simulink model "Model"  (R2023b)
settings: Solver=FixedStepAuto  StartTime=0.0  StopTime=10  FixedStep=0.002  RelTol=1e-3
undefined symbols (not defined in the file or in its folder): K, X, Y, Z
libraries: sm_lib x47, nesl_utility x15, simulink x2, slpidlib x2
(part 3 of 4)

== matlab function Model/右腿VMC ==
  data: phi_1 input; phi_4 input; F input; T1 output; T2 output; Tp input
function [T1,T2]= fcn(phi_1,phi_4,F,Tp)

l_1=0.15;
l_2=0.27;
l_3=0.27;
l_4=0.15;
l_5=0.15;

J11=(2*(l_1*cos(phi_1) + (2*l_2*cos(2*atan(((4*l_2^2*(l_1*sin(phi_1) - l_4*sin(phi_4))^2 - ((l_1*sin(phi_1) - l_4*sin(phi_4))^2 + (l_5 - l_1*cos(phi_1) + l_4*cos(phi_4))^2 + l_2^2 - l_3^2)^2 + 4*l_2^2*(l_5 - l_1*cos(phi_1) + l_4*cos(phi_4))^2)^(1/2) - 2*l_2*(l_1*sin(phi_1) - l_4*sin(phi_4)))/((l_1*sin(phi_1) - l_4*sin(phi_4))^2 + (l_5 - l_1*cos(phi_1) + l_4*cos(phi_4))^2 + l_2^2 - l_3^2 + 2*l_2*(l_5 - l_1*cos(phi_1) + l_4*cos(phi_4)))))*(((8*l_1*l_2^2*cos(phi_1)*(l_1*sin(phi_1) - l_4*sin(phi_4)) - 2*(2*l_1*cos(phi_1)*(l_1*sin(phi_1) - l_4*sin(phi_4)) + 2*l_1*sin(phi_1)*(l_5 - l_1*cos(phi_1) + l_4*cos(phi_4)))*((l_1*sin(phi_1) - l_4*sin(phi_4))^2 + (l_5 - l_1*cos(phi_1) + l_4*cos(phi_4))^2 + l_2^2 - l_3^2) + 8*l_1*l_2^2*sin(phi_1)*(l_5 - l_1*cos(phi_1) + l_4*cos(phi_4)))/(2*(4*l_2^2*(l_1*sin(phi_1) - l_4*sin(phi_4))^2 - ((l_1*sin(phi_1) - l_4*sin(phi_4))^2 + (l_5 - l_1*cos(phi_1) + l_4*cos(phi_4))^2 + l_2^2 - l_3^2)^2 + 4*l_2^2*(l_5 - l_1*cos(phi_1) + l_4*cos(phi_4))^2)^(1/2)) - 2*l_1*l_2*cos(phi_1))/((l_1*sin(phi_1) - l_4*sin(phi_4))^2 + (l_5 - l_1*cos(phi_1) + l_4*cos(phi_4))^2 + l_2^2 - l_3^2 + 2*l_2*(l_5 - l_1*cos(phi_1) + l_4*cos(phi_4))) - (((4*l_2^2*(l_1*sin(phi_1) - l_4*sin(phi_4))^2 - ((l_1*sin(phi_1) - l_4*sin(phi_4))^2 + (l_5 - l_1*cos(phi_1) + l_4*cos(phi_4))^2 + l_2^2 - l_3^2)^2 + 4*l_2^2*(l_5 - l_1*cos(phi_1) + l_4*cos(phi_4))^2)^(1/2) - 2*l_2*(l_1*sin(phi_1) - l_4*sin(phi_4)))*(2*l_1*l_2*sin(phi_1) + 2*l_1*cos(phi_1)*(l_1*sin(phi_1) - l_4*sin(phi_4)) + 2*l_1*sin(phi_1)*(l_5 - l_1*cos(phi_1) + l_4*cos(phi_4))))/((l_1*sin(phi_1) - l_4*sin(phi_4))^2 + (l_5 - l_1*cos(phi_1) + l_4*cos(phi_4))^2 + l_2^2 - l_3^2 + 2*l_2*(l_5 - l_1*cos(phi_1) + l_4*cos(phi_4)))^2))/(((4*l_2^2*(l_1*sin(phi_1) - l_4*sin(phi_4))^2 - ((l_1*sin(phi_1) - l_4*sin(phi_4))^2 + (l_5 - l_1*cos(phi_1) + l_4*cos(phi_4))^2 + l_2^2 - l_3^2)^2 + 4*l_2^2*(l_5 - l_1*cos(phi_1) + l_4*cos(phi_4))^2)^(1/2) - 2*l_2*(l_1*sin(phi_1) - l_4*sin(phi_4)))^2/((l_1*sin(phi_1) - l_4*sin(phi_4))^2 + (l_5 - l_1*cos(phi_1) + l_4*cos(phi_4))^2 + l_2^2 - l_3^2 + 2*l_2*(l_5 - l_1*cos(phi_1) + l_4*cos(phi_4)))^2 + 1))*(l_2*sin(2*atan(((4*l_2^2*(l_1*sin(phi_1) - l_4*sin(phi_4))^2 - ((l_1*sin(phi_1) - l_4*sin(phi_4))^2 + (l_5 - l_1*cos(phi_1) + l_4*cos(phi_4))^2 + l_2^2 - l_3^2)^2 + 4*l_2^2*(l_5 - l_1*cos(phi_1) + l_4*cos(phi_4))^2)^(1/2) - 2*l_2*(l_1*sin(phi_1) - l_4*sin(phi_4)))/((l_1*sin(phi_1) - l_4*sin(phi_4))^2 + (l_5 - l_1*cos(phi_1) + l_4*cos(phi_4))^2 + l_2^2 - l_3^2 + 2*l_2*(l_5 - l_1*cos(phi_1) + l_4*cos(phi_4))))) + l_1*sin(phi_1)) - 2*(l_1*sin(phi_1) + (2*l_2*sin(2*atan(((4*l_2^2*(l_1*sin(phi_1) - l_4*sin(phi_4))^2 - ((l_1*sin(phi_1) - l_4*sin(phi_4))^2 + (l_5 - l_1*cos(phi_1) + l_4*cos(phi_4))^2 + l_2^2 - l_3^2)^2 + 4*l_2^2*(l_5 - l_1*cos(phi_1) + l_4*cos(phi_4))^2)^(1/2) - 2*l_2*(l_1*sin(phi_1) - l_4*sin(phi_4)))/((l_1*sin(phi_1) - l_4*sin(phi_4))^2 + (l_5 - l_1*cos(phi_1) + l_4*cos(phi_4))^2 + l_2^2 - l_3^2 + 2*l_2*(l_5 - l_1*cos(phi_1) + l_4*cos(phi_4)))))*(((8*l_1*l_2^2*cos(phi_1)*(l_1*sin(phi_1) - l_4*sin(phi_4)) - 2*(2*l_1*cos(phi_1)*(l_1*sin(phi_1) - l_4*sin(phi_4)) + 2*l_1*sin(phi_1)*(l_5 - l_1*cos(phi_1) + l_4*cos(phi_4)))*((l_1*sin(phi_1) - l_4*sin(phi_4))^2 + (l_5 - l_1*cos(phi_1) + l_4*cos(phi_4))^2 + l_2^2 - l_3^2) + 8*l_1*l_2^2*sin(phi_1)*(l_5 - l_1*cos(phi_1) + l_4*cos(phi_4)))/(2*(4*l_2^2*(l_1*sin(phi_1) - l_4*sin(phi_4))^2 - ((l_1*sin(phi_1) - l_4*sin(phi_4))^2 + (l_5 - l_1*cos(phi_1) + l_4*cos(phi_4))^2 + l_2^2 - l_3^2)^2 + 4*l_2^2*(l_5 - l_1*cos(phi_1) + l_4*cos(phi_4))^2)^(1/2)) - 2*l_1*l_2*cos(phi_1))/((l_1*sin(phi_1) - l_4*sin(phi_4))^2 + (l_5 - l_1*cos(phi_1) + l_4*cos(phi_4))^2 + l_2^2 - l_3^2 + 2*l_2*(l_5 - l_1*cos(phi_1) + l_4*cos(phi_4))) - (((4*l_2^2*(l_1*sin(phi_1) - l_4*sin(phi_4))^2 - ((l_1*sin(phi_1) - l_4*sin(phi_4))^2 + (l_5 - l_1*cos(phi_1) + l_4*cos(phi_4))^2 + l_2^2 - l_3^2)^2 + 4*l_2^2*(l_5 - l_1*cos(phi_1) + l_4*cos(phi_4))^2)^(1/2) - 2*l_2*(l_1*sin(phi_1) - l_4*sin(phi_4)))*(2*l_1*l_2*sin(phi_1) + 2*l_1*cos(phi_1)*(l_1*sin(phi_1) - l_4*sin(phi_4)) + 2*l_1*sin(phi_1)*(l_5 - l_1*cos(phi_1) + l_4*cos(phi_4))))/((l_1*sin(phi_1) - l_4*sin(phi_4))^2 + (l_5 - l_1*cos(phi_1) + l_4*cos(phi_4))^2 + l_2^2 - l_3^2 + 2*l_2*(l_5 - l_1*cos(phi_1) + l_4*cos(phi_4)))^2))/(((4*l_2^2*(l_1*sin(phi_1) - l_4*sin(phi_4))^2 - ((l_1*sin(phi_1) - l_4*sin(phi_4))^2 + (l_5 - l_1*cos(phi_1) + l_4*cos(phi_4))^2 + l_2^2 - l_3^2)^2 + 4*l_2^2*(l_5 - l_1*cos(phi_1) + l_4*cos(phi_4))^2)^(1/2) - 2*l_2*(l_1*sin(phi_1) - l_4*sin(phi_4)))^2/((l_1*sin(phi_1) - l_4*sin(phi_4))^2 + (l_5 - l_1*cos(phi_1) + l_4*cos(phi_4))^2 + l_2^2 - l_3^2 + 2*l_2*(l_5 - l_1*cos(phi_1) + l_4*cos(phi_4)))^2 + 1))*(l_2*cos(2*atan(((4*l_2^2*(l_1*sin(phi_1) - l_4*sin(phi_4))^2 - ((l_1*sin(phi_1) - l_4*sin(phi_4))^2 + (l_5 - l_1*cos(phi_1) + l_4*cos(phi_4))^2 + l_2^2 - l_3^2)^2 + 4*l_2^2*(l_5 - l_1*cos(phi_1) + l_4*cos(phi_4))^2)^(1/2) - 2*l_2*(l_1*sin(phi_1) - l_4*sin(phi_4)))/((l_1*sin(phi_1) - l_4*sin(phi_4))^2 + (l_5 - l_1*cos(phi_1) + l_4*cos(phi_4))^2 + l_2^2 - l_3^2 + 2*l_2*(l_5 - l_1*cos(phi_1) + l_4*cos(phi_4))))) - l_5/2 + l_1*cos(phi_1)))/(2*((l_2*sin(2*atan(((4*l_2^2*(l_1*sin(phi_1) - l_4*sin(phi_4))^2 - ((l_1*sin(phi_1) - l_4*sin(phi_4))^2 + (l_5 - l_1*cos(phi_1) + l_4*cos(phi_4))^2 + l_2^2 - l_3^2)^2 + 4*l_2^2*(l_5 - l_1*cos(phi_1) + l_4*cos(phi_4))^2)^(1/2) - 2*l_2*(l_1*sin(phi_1) - l_4*sin(phi_4)))/((l_1*sin(phi_1) - l_4*sin(phi_4))^2 + (l_5 - l_1*cos(phi_1) + l_4*cos(phi_4))^2 + l_2^2 - l_3^2 + 2*l_2*(l_5 - l_1*cos(phi_1) + l_4*cos(phi_4))))) + l_1*sin(phi_1))^2 + (l_2*cos(2*atan(((4*l_2^2*(l_1*sin(phi_1) - l_4*sin(phi_4))^2 - ((l_1*sin(phi_1) - l_4*sin(phi_4))^2 + (l_5 - l_1*cos(phi_1) + l_4*cos(phi_4))^2 + l_2^2 - l_3^2)^2 + 4*l_2^2*(l_5 - l_1*cos(phi_1) + l_4*cos(phi_4))^2)^(1/2) - 2*l_2*(l_1*sin(phi_1) - l_4*sin(phi_4)))/((l_1*sin(phi_1) - l_4*sin(phi_4))^2 + (l_5 - l_1*cos(phi_1) + l_4*cos(phi_4))^2 + l_2^2 - l_3^2 + 2*l_2*(l_5 - l_1*cos(phi_1) + l_4*cos(phi_4))))) - l_5/2 + l_1*cos(phi_1))^2)^(1/2));
J12=((4*l_2*sin(2*atan(((4*l_2^2*(l_1*sin(phi_1) - l_4*sin(phi_4))^2 - ((l_1*sin(phi_1) - l_4*sin(phi_4))^2 + (l_5 - l_1*cos(phi_1) + l_4*cos(phi_4))^2 + l_2^2 - l_3^2)^2 + 4*l_2^2*(l_5 - l_1*cos(phi_1) + l_4*cos(phi_4))^2)^(1/2) - 2*l_2*(l_1*sin(phi_1) - l_4*sin(phi_4)))/((l_1*sin(phi_1) - l_4*sin(phi_4))^2 + (l_5 - l_1*cos(phi_1) + l_4*cos(phi_4))^2 + l_2^2 - l_3^2 + 2*l_2*(l_5 - l_1*cos(phi_1) + l_4*cos(phi_4)))))*(((8*l_2^2*l_4*cos(phi_4)*(l_1*sin(phi_1) - l_4*sin(phi_4)) - 2*(2*l_4*cos(phi_4)*(l_1*sin(phi_1) - l_4*sin(phi_4)) + 2*l_4*sin(phi_4)*(l_5 - l_1*cos(phi_1) + l_4*cos(phi_4)))*((l_1*sin(phi_1) - l_4*sin(phi_4))^2 + (l_5 - l_1*cos(phi_1) + l_4*cos(phi_4))^2 + l_2^2 - l_3^2) + 8*l_2^2*l_4*sin(phi_4)*(l_5 - l_1*cos(phi_1) + l_4*cos(phi_4)))/(2*(4*l_2^2*(l_1*sin(phi_1) - l_4*sin(phi_4))^2 - ((l_1*sin(phi_1) - l_4*sin(phi_4))^2 + (l_5 - l_1*cos(phi_1) + l_4*cos(phi_4))^2 + l_2^2 - l_3^2)^2 + 4*l_2^2*(l_5 - l_1*cos(phi_1) + l_4*cos(phi_4))^2)^(1/2)) - 2*l_2*l_4*cos(phi_4))/((l_1*sin(phi_1) - l_4*sin(phi_4))^2 + (l_5 - l_1*cos(phi_1) + l_4*cos(phi_4))^2 + l_2^2 - l_3^2 + 2*l_2*(l_5 - l_1*cos(phi_1) + l_4*cos(phi_4))) - (((4*l_2^2*(l_1*sin(phi_1) - l_4*sin(phi_4))^2 - ((l_1*sin(phi_1) - l_4*sin(phi_4))^2 + (l_5 - l_1*cos(phi_1) + l_4*cos(phi_4))^2 + l_2^2 - l_3^2)^2 + 4*l_2^2*(l_5 - l_1*cos(phi_1) + l_4*cos(phi_4))^2)^(1/2) - 2*l_2*(l_1*sin(phi_1) - l_4*sin(phi_4)))*(2*l_2*l_4*sin(phi_4) + 2*l_4*cos(phi_4)*(l_1*sin(phi_1) - l_4*sin(phi_4)) + 2*l_4*sin(phi_4)*(l_5 - l_1*cos(phi_1) + l_4*cos(phi_4))))/((l_1*sin(phi_1) - l_4*sin(phi_4))^2 + (l_5 - l_1*cos(phi_1) + l_4*cos(phi_4))^2 + l_2^2 - l_3^2 + 2*l_2*(l_5 - l_1*cos(phi_1) + l_4*cos(phi_4)))^2)*(l_2*cos(2*atan(((4*l_2^2*(l_1*sin(phi_1) - l_4*sin(phi_4))^2 - ((l_1*sin(phi_1) - l_4*sin(phi_4))^2 + (l_5 - l_1*cos(phi_1) + l_4*cos(phi_4))^2 + l_2^2 - l_3^2)^2 + 4*l_2^2*(l_5 - l_1*cos(phi_1) + l_4*cos(phi_4))^2)^(1/2) - 2*l_2*(l_1*sin(phi_1) - l_4*sin(phi_4)))/((l_1*sin(phi_1) - l_4*sin(phi_4))^2 + (l_5 - l_1*cos(phi_1) + l_4*cos(phi_4))^2 + l_2^2 - l_3^2 + 2*l_2*(l_5 - l_1*cos(phi_1) + l_4*cos(phi_4))))) - l_5/2 + l_1*cos(phi_1)))/(((4*l_2^2*(l_1*sin(phi_1) - l_4*sin(phi_4))^2 - ((l_1*sin(phi_1) - l_4*sin(phi_4))^2 + (l_5 - l_1*cos(phi_1) + l_4*cos(phi_4))^2 + l_2^2 - l_3^2)^2 + 4*l_2^2*(l_5 - l_1*cos(phi_1) + l_4*cos(phi_4))^2)^(1/2) - 2*l_2*(l_1*sin(phi_1) - l_4*sin(phi_4)))^2/((l_1*sin(phi_1) - l_4*sin(phi_4))^2 + (l_5 - l_1*cos(phi_1) + l_4*cos(phi_4))^2 + l_2^2 - l_3^2 + 2*l_2*(l_5 - l_1*cos(phi_1) + l_4*cos(phi_4)))^2 + 1) - (4*l_2*cos(2*atan(((4*l_2^2*(l_1*sin(phi_1) - l_4*sin(phi_4))^2 - ((l_1*sin(phi_1) - l_4*sin(phi_4))^2 + (l_5 - l_1*cos(phi_1) + l_4*cos(phi_4))^2 + l_2^2 - l_3^2)^2 + 4*l_2^2*(l_5 - l_1*cos(phi_1) + l_4*cos(phi_4))^2)^(1/2) - 2*l_2*(l_1*sin(phi_1) - l_4*sin(phi_4)))/((l_1*sin(phi_1) - l_4*sin(phi_4))^2 + (l_5 - l_1*cos(phi_1) + l_4*cos(phi_4))^2 + l_2^2 - l_3^2 + 2*l_2*(l_5 - l_1*cos(phi_1) + l_4*cos(phi_4)))))*(l_2*sin(2*atan(((4*l_2^2*(l_1*sin(phi_1) - l_4*sin(phi_4))^2 - ((l_1*sin(phi_1) - l_4*sin(phi_4))^2 + (l_5 - l_1*cos(phi_1) + l_4*cos(phi_4))^2 + l_2^2 - l_3^2)^2 + 4*l_2^2*(l_5 - l_1*cos(phi_1) + l_4*cos(phi_4))^2)^(1/2) - 2*l_2*(l_1*sin(phi_1) - l_4*sin(phi_4)))/((l_1*sin(phi_1) - l_4*sin(phi_4))^2 + (l_5 - l_1*cos(phi_1) + l_4*cos(phi_4))^2 + l_2^2 - l_3^2 + 2*l_2*(l_5 - l_1*cos(phi_1) + l_4*cos(phi_4))))) + l_1*sin(phi_1))*(((8*l_2^2*l_4*cos(phi_4)*(l_1*sin(phi_1) - l_4*sin(phi_4)) - 2*(2*l_4*cos(phi_4)*(l_1*sin(phi_1) - l_4*sin(phi_4)) + 2*l_4*sin(phi_4)*(l_5 - l_1*cos(phi_1) + l_4*cos(phi_4)))*((l_1*sin(phi_1) - l_4*sin(phi_4))^2 + (l_5 - l_1*cos(phi_1) + l_4*cos(phi_4))^2 + l_2^2 - l_3^2) + 8*l_2^2*l_4*sin(phi_4)*(l_5 - l_1*cos(phi_1) + l_4*cos(phi_4)))/(2*(4*l_2^2*(l_1*sin(phi_1) - l_4*sin(phi_4))^2 - ((l_1*sin(phi_1) - l_4*sin(phi_4))^2 + (l_5 - l_1*cos(phi_1) + l_4*cos(phi_4))^2 + l_2^2 - l_3^2)^2 + 4*l_2^2*(l_5 - l_1*cos(phi_1) + l_4*cos(phi_4))^2)^(1/2)) - 2*l_2*l_4*cos(phi_4))/((l_1*sin(phi_1) - l_4*sin(phi_4))^2 + (l_5 - l_1*cos(phi_1) + l_4*cos(phi_4))^2 + l_2^2 - l_3^2 + 2*l_2*(l_5 - l_1*cos(phi_1) + l_4*cos(phi_4))) - (((4*l_2^2*(l_1*sin(phi_1) - l_4*sin(phi_4))^2 - ((l_1*sin(phi_1) - l_4*sin(phi_4))^2 + (l_5 - l_1*cos(phi_1) + l_4*cos(phi_4))^2 + l_2^2 - l_3^2)^2 + 4*l_2^2*(l_5 - l_1*cos(phi_1) + l_4*cos(phi_4))^2)^(1/2) - 2*l_2*(l_1*sin(phi_1) - l_4*sin(phi_4)))*(2*l_2*l_4*sin(phi_4) + 2*l_4*cos(phi_4)*(l_1*sin(phi_1) - l_4*sin(phi_4)) + 2*l_4*sin(phi_4)*(l_5 - l_1*cos(phi_1) + l_4*cos(phi_4))))/((l_1*sin(phi_1) - l_4*sin(phi_4))^2 + (l_5 - l_1*cos(phi_1) + l_4*cos(phi_4))^2 + l_2^2 - l_3^2 + 2*l_2*(l_5 - l_1*cos(phi_1) + l_4*cos(phi_4)))^2))/(((4*l_2^2*(l_1*sin(phi_1) - l_4*sin(phi_4))^2 - ((l_1*sin(phi_1) - l_4*sin(phi_4))^2 + (l_5 - l_1*cos(phi_1) + l_4*cos(phi_4))^2 + l_2^2 - l_3^2)^2 + 4*l_2^2*(l_5 - l_1*cos(phi_1) + l_4*cos(phi_4))^2)^(1/2) - 2*l_2*(l_1*sin(phi_1) - l_4*sin(phi_4)))^2/((l_1*sin(phi_1) - l_4*sin(phi_4))^2 + (l_5 - l_1*cos(phi_1) + l_4*cos(phi_4))^2 + l_2^2 - l_3^2 + 2*l_2*(l_5 - l_1*cos(phi_1) + l_4*cos(phi_4)))^2 + 1))/(2*((l_2*sin(2*atan(((4*l_2^2*(l_1*sin(phi_1) - l_4*sin(phi_4))^2 - ((l_1*sin(phi_1) - l_4*sin(phi_4))^2 + (l_5 - l_1*cos(phi_1) + l_4*cos(phi_4))^2 + l_2^2 - l_3^2)^2 + 4*l_2^2*(l_5 - l_1*cos(phi_1) + l_4*cos(phi_4))^2)^(1/2) - 2*l_2*(l_1*sin(phi_1) - l_4*sin(phi_4)))/((l_1*sin(phi_1) - l_4*sin(phi_4))^2 + (l_5 - l_1*cos(phi_1) + l_4*cos(phi_4))^2 + l_2^2 - l_3^2 + 2*l_2*(l_5 - l_1*cos(phi_1) + l_4*cos(phi_4))))) + l_1*sin(phi_1))^2 + (l_2*cos(2*atan(((4*l_2^2*(l_1*sin(phi_1) - l_4*sin(phi_4))^2 - ((l_1*sin(phi_1) - l_4*sin(phi_4))^2 + (l_5 - l_1*cos(phi_1) + l_4*cos(phi_4))^2 + l_2^2 - l_3^2)^2 + 4*l_2^2*(l_5 - l_1*cos(phi_1) + l_4*cos(phi_4))^2)^(1/2) - 2*l_2*(l_1*sin(phi_1) - l_4*sin(phi_4)))/((l_1*sin(phi_1) - l_4*sin(phi_4))^2 + (l_5 - l_1*cos(phi_1) + l_4*cos(phi_4))^2 + l_2^2 - l_3^2 + 2*l_2*(l_5 - l_1*cos(phi_1) + l_4*cos(phi_4))))) - l_5/2 + l_1*cos(phi_1))^2)^(1/2));
J21=((l_1*sin(phi_1) + (2*l_2*sin(2*atan(((4*l_2^2*(l_1*sin(phi_1) - l_4*sin(phi_4))^2 - ((l_1*sin(phi_1) - l_4*sin(phi_4))^2 + (l_5 - l_1*cos(phi_1) + l_4*cos(phi_4))^2 + l_2^2 - l_3^2)^2 + 4*l_2^2*(l_5 - l_1*cos(phi_1) + l_4*cos(phi_4))^2)^(1/2) - 2*l_2*(l_1*sin(phi_1) - l_4*sin(phi_4)))/((l_1*sin(phi_1) - l_4*sin(phi_4))^2 + (l_5 - l_1*cos(phi_1) + l_4*cos(phi_4))^2 + l_2^2 - l_3^2 + 2*l_2*(l_5 - l_1*cos(phi_1) + l_4*cos(phi_4)))))*(((8*l_1*l_2^2*cos(phi_1)*(l_1*sin(phi_1) - l_4*sin(phi_4)) - 2*(2*l_1*cos(phi_1)*(l_1*sin(phi_1) - l_4*sin(phi_4)) + 2*l_1*sin(phi_1)*(l_5 - l_1*cos(phi_1) + l_4*cos(phi_4)))*((l_1*sin(phi_1) - l_4*sin(phi_4))^2 + (l_5 - l_1*cos(phi_1) + l_4*cos(phi_4))^2 + l_2^2 - l_3^2) + 8*l_1*l_2^2*sin(phi_1)*(l_5 - l_1*cos(phi_1) + l_4*cos(phi_4)))/(2*(4*l_2^2*(l_1*sin(phi_1) - l_4*sin(phi_4))^2 - ((l_1*sin(phi_1) - l_4*sin(phi_4))^2 + (l_5 - l_1*cos(phi_1) + l_4*cos(phi_4))^2 + l_2^2 - l_3^2)^2 + 4*l_2^2*(l_5 - l_1*cos(phi_1) + l_4*cos(phi_4))^2)^(1/2)) - 2*l_1*l_2*cos(phi_1))/((l_1*sin(phi_1) - l_4*sin(phi_4))^2 + (l_5 - l_1*cos(phi_1) + l_4*cos(phi_4))^2 + l_2^2 - l_3^2 + 2*l_2*(l_5 - l_1*cos(phi_1) + l_4*cos(phi_4))) - (((4*l_2^2*(l_1*sin(phi_1) - l_4*sin(phi_4))^2 - ((l_1*sin(phi_1) - l_4*sin(phi_4))^2 + (l_5 - l_1*cos(phi_1) + l_4*cos(phi_4))^2 + l_2^2 - l_3^2)^2 + 4*l_2^2*(l_5 - l_1*cos(phi_1) + l_4*cos(phi_4))^2)^(1/2) - 2*l_2*(l_1*sin(phi_1) - l_4*sin(phi_4)))*(2*l_1*l_2*sin(phi_1) + 2*l_1*cos(phi_1)*(l_1*sin(phi_1) - l_4*sin(phi_4)) + 2*l_1*sin(phi_1)*(l_5 - l_1*cos(phi_1) + l_4*cos(phi_4))))/((l_1*sin(phi_1) - l_4*sin(phi_4))^2 + (l_5 - l_1*cos(phi_1) + l_4*cos(phi_4))^2 + l_2^2 - l_3^2 + 2*l_2*(l_5 - l_1*cos(phi_1) + l_4*cos(phi_4)))^2))/(((4*l_2^2*(l_1*sin(phi_1) - l_4*sin(phi_4))^2 - ((l_1*sin(phi_1) - l_4*sin(phi_4))^2 + (l_5 - l_1*cos(phi_1) + l_4*cos(phi_4))^2 + l_2^2 - l_3^2)^2 + 4*l_2^2*(l_5 - l_1*cos(phi_1) + l_4*cos(phi_4))^2)^(1/2) - 2*l_2*(l_1*sin(phi_1) - l_4*sin(phi_4)))^2/((l_1*sin(phi_1) - l_4*sin(phi_4))^2 + (l_5 - l_1*cos(phi_1) + l_4*cos(phi_4))^2 + l_2^2 - l_3^2 + 2*l_2*(l_5 - l_1*cos(phi_1) + l_4*cos(phi_4)))^2 + 1))/((l_2*sin(2*atan(((4*l_2^2*(l_1*sin(phi_1) - l_4*sin(phi_4))^2 - ((l_1*sin(phi_1) - l_4*sin(phi_4))^2 + (l_5 - l_1*cos(phi_1) + l_4*cos(phi_4))^2 + l_2^2 - l_3^2)^2 + 4*l_2^2*(l_5 - l_1*cos(phi_1) + l_4*cos(phi_4))^2)^(1/2) - 2*l_2*(l_1*sin(phi_1) - l_4*sin(phi_4)))/((l_1*sin(phi_1) - l_4*sin(phi_4))^2 + (l_5 - l_1*cos(phi_1) + l_4*cos(phi_4))^2 + l_2^2 - l_3^2 + 2*l_2*(l_5 - l_1*cos(phi_1) + l_4*cos(phi_4))))) + l_1*sin(phi_1))^2 + (l_2*cos(2*atan(((4*l_2^2*(l_1*sin(phi_1) - l_4*sin(phi_4))^2 - ((l_1*sin(phi_1) - l_4*sin(phi_4))^2 + (l_5 - l_1*cos(phi_1) + l_4*cos(phi_4))^2 + l_2^2 - l_3^2)^2 + 4*l_2^2*(l_5 - l_1*cos(phi_1) + l_4*cos(phi_4))^2)^(1/2) - 2*l_2*(l_1*sin(phi_1) - l_4*sin(phi_4)))/((l_1*sin(phi_1) - l_4*sin(phi_4))^2 + (l_5 - l_1*cos(phi_1) + l_4*cos(phi_4))^2 + l_2^2 - l_3^2 + 2*l_2*(l_5 - l_1*cos(phi_1) + l_4*cos(phi_4))))) - l_5/2 + l_1*cos(phi_1))^2)^(1/2) + ((2*(l_1*cos(phi_1) + (2*l_2*cos(2*atan(((4*l_2^2*(l_1*sin(phi_1) - l_4*sin(phi_4))^2 - ((l_1*sin(phi_1) - l_4*sin(phi_4))^2 + (l_5 - l_1*cos(phi_1) + l_4*cos(phi_4))^2 + l_2^2 - l_3^2)^2 + 4*l_2^2*(l_5 - l_1*cos(phi_1) + l_4*cos(phi_4))^2)^(1/2) - 2*l_2*(l_1*sin(phi_1) - l_4*sin(phi_4)))/((l_1*sin(phi_1) - l_4*sin(phi_4))^2 + (l_5 - l_1*cos(phi_1) + l_4*cos(phi_4))^2 + l_2^2 - l_3^2 + 2*l_2*(l_5 - l_1*cos(phi_1) + l_4*cos(phi_4)))))*(((8*l_1*l_2^2*cos(phi_1)*(l_1*sin(phi_1) - l_4*sin(phi_4)) - 2*(2*l_1*cos(phi_1)*(l_1*sin(phi_1) - l_4*sin(phi_4)) + 2*l_1*sin(phi_1)*(l_5 - l_1*cos(phi_1) + l_4*cos(phi_4)))*((l_1*sin(phi_1) - l_4*sin(phi_4))^2 + (l_5 - l_1*cos(phi_1) + l_4*cos(phi_4))^2 + l_2^2 - l_3^2) + 8*l_1*l_2^2*sin(phi_1)*(l_5 - l_1*cos(phi_1) + l_4*cos(phi_4)))/(2*(4*l_2^2*(l_1*sin(phi_1) - l_4*sin(phi_4))^2 - ((l_1*sin(phi_1) - l_4*sin(phi_4))^2 + (l_5 - l_1*cos(phi_1) + l_4*cos(phi_4))^2 + l_2^2 - l_3^2)^2 + 4*l_2^2*(l_5 - l_1*cos(phi_1) + l_4*cos(phi_4))^2)^(1/2)) - 2*l_1*l_2*cos(phi_1))/((l_1*sin(phi_1) - l_4*sin(phi_4))^2 + (l_5 - l_1*cos(phi_1) + l_4*cos(phi_4))^2 + l_2^2 - l_3^2 + 2*l_2*(l_5 - l_1*cos(phi_1) + l_4*cos(phi_4))) - (((4*l_2^2*(l_1*sin(phi_1) - l_4*sin(phi_4))^2 - ((l_1*sin(phi_1) - l_4*sin(phi_4))^2 + (l_5 - l_1*cos(phi_1) + l_4*cos(phi_4))^2 + l_2^2 - l_3^2)^2 + 4*l_2^2*(l_5 - l_1*cos(phi_1) + l_4*cos(phi_4))^2)^(1/2) - 2*l_2*(l_1*sin(phi_1) - l_4*sin(phi_4)))*(2*l_1*l_2*sin(phi_1) + 2*l_1*cos(phi_1)*(l_1*sin(phi_1) - l_4*sin(phi_4)) + 2*l_1*sin(phi_1)*(l_5 - l_1*cos(phi_1) + l_4*cos(phi_4))))/((l_1*sin(phi_1) - l_4*sin(phi_4))^2 + (l_5 - l_1*cos(phi_1) + l_4*cos(phi_4))^2 + l_2^2 - l_3^2 + 2*l_2*(l_5 - l_1*cos(phi_1) + l_4*cos(phi_4)))^2))/(((4*l_2^2*(l_1*sin(phi_1) - l_4*sin(phi_4))^2 - ((l_1*sin(phi_1) - l_4*sin(phi_4))^2 + (l_5 - l_1*cos(phi_1) + l_4*cos(phi_4))^2 + l_2^2 - l_3^2)^2 + 4*l_2^2*(l_5 - l_1*cos(phi_1) + l_4*cos(phi_4))^2)^(1/2) - 2*l_2*(l_1*sin(phi_1) - l_4*sin(phi_4)))^2/((l_1*sin(phi_1) - l_4*sin(phi_4))^2 + (l_5 - l_1*cos(phi_1) + l_4*cos(phi_4))^2 + l_2^2 - l_3^2 + 2*l_2*(l_5 - l_1*cos(phi_1) + l_4*cos(phi_4)))^2 + 1))*(l_2*sin(2*atan(((4*l_2^2*(l_1*sin(phi_1) - l_4*sin(phi_4))^2 - ((l_1*sin(phi_1) - l_4*sin(phi_4))^2 + (l_5 - l_1*cos(phi_1) + l_4*cos(phi_4))^2 + l_2^2 - l_3^2)^2 + 4*l_2^2*(l_5 - l_1*cos(phi_1) + l_4*cos(phi_4))^2)^(1/2) - 2*l_2*(l_1*sin(phi_1) - l_4*sin(phi_4)))/((l_1*sin(phi_1) - l_4*sin(phi_4))^2 + (l_5 - l_1*cos(phi_1) + l_4*cos(phi_4))^2 + l_2^2 - l_3^2 + 2*l_2*(l_5 - l_1*cos(phi_1) + l_4*cos(phi_4))))) + l_1*sin(phi_1)) - 2*(l_1*sin(phi_1) + (2*l_2*sin(2*atan(((4*l_2^2*(l_1*sin(phi_1) - l_4*sin(phi_4))^2 - ((l_1*sin(phi_1) - l_4*sin(phi_4))^2 + (l_5 - l_1*cos(phi_1) + l_4*cos(phi_4))^2 + l_2^2 - l_3^2)^2 + 4*l_2^2*(l_5 - l_1*cos(phi_1) + l_4*cos(phi_4))^2)^(1/2) - 2*l_2*(l_1*sin(phi_1) - l_4*sin(phi_4)))/((l_1*sin(phi_1) - l_4*sin(phi_4))^2 + (l_5 - l_1*cos(phi_1) + l_4*cos(phi_4))^2 + l_2^2 - l_3^2 + 2*l_2*(l_5 - l_1*cos(phi_1) + l_4*cos(phi_4)))))*(((8*l_1*l_2^2*cos(phi_1)*(l_1*sin(phi_1) - l_4*sin(phi_4)) - 2*(2*l_1*cos(phi_1)*(l_1*sin(phi_1) - l_4*sin(phi_4)) + 2*l_1*sin(phi_1)*(l_5 - l_1*cos(phi_1) + l_4*cos(phi_4)))*((l_1*sin(phi_1) - l_4*sin(phi_4))^2 + (l_5 - l_1*cos(phi_1) + l_4*cos(phi_4))^2 + l_2^2 - l_3^2) + 8*l_1*l_2^2*sin(phi_1)*(l_5 - l_1*cos(phi_1) + l_4*cos(phi_4)))/(2*(4*l_2^2*(l_1*sin(phi_1) - l_4*sin(phi_4))^2 - ((l_1*sin(phi_1) - l_4*sin(phi_4))^2 + (l_5 - l_1*cos(phi_1) + l_4*cos(phi_4))^2 + l_2^2 - l_3^2)^2 + 4*l_2^2*(l_5 - l_1*cos(phi_1) + l_4*cos(phi_4))^2)^(1/2)) - 2*l_1*l_2*cos(phi_1))/((l_1*sin(phi_1) - l_4*sin(phi_4))^2 + (l_5 - l_1*cos(phi_1) + l_4*cos(phi_4))^2 + l_2^2 - l_3^2 + 2*l_2*(l_5 - l_1*cos(phi_1) + l_4*cos(phi_4))) - (((4*l_2^2*(l_1*sin(phi_1) - l_4*sin(phi_4))^2 - ((l_1*sin(phi_1) - l_4*sin(phi_4))^2 + (l_5 - l_1*cos(phi_1) + l_4*cos(phi_4))^2 + l_2^2 - l_3^2)^2 + 4*l_2^2*(l_5 - l_1*cos(phi_1) + l_4*cos(phi_4))^2)^(1/2) - 2*l_2*(l_1*sin(phi_1) - l_4*sin(phi_4)))*(2*l_1*l_2*sin(phi_1) + 2*l_1*cos(phi_1)*(l_1*sin(phi_1) - l_4*sin(phi_4)) + 2*l_1*sin(phi_1)*(l_5 - l_1*cos(phi_1) + l_4*cos(phi_4))))/((l_1*sin(phi_1) - l_4*sin(phi_4))^2 + (l_5 - l_1*cos(phi_1) + l_4*cos(phi_4))^2 + l_2^2 - l_3^2 + 2*l_2*(l_5 - l_1*cos(phi_1) + l_4*cos(phi_4)))^2))/(((4*l_2^2*(l_1*sin(phi_1) - l_4*sin(phi_4))^2 - ((l_1*sin(phi_1) - l_4*sin(phi_4))^2 + (l_5 - l_1*cos(phi_1) + l_4*cos(phi_4))^2 + l_2^2 - l_3^2)^2 + 4*l_2^2*(l_5 - l_1*cos(phi_1) + l_4*cos(phi_4))^2)^(1/2) - 2*l_2*(l_1*sin(phi_1) - l_4*sin(phi_4)))^2/((l_1*sin(phi_1) - l_4*sin(phi_4))^2 + (l_5 - l_1*cos(phi_1) + l_4*cos(phi_4))^2 + l_2^2 - l_3^2 + 2*l_2*(l_5 - l_1*cos(phi_1) + l_4*cos(phi_4)))^2 + 1))*(l_2*cos(2*atan(((4*l_2^2*(l_1*sin(phi_1) - l_4*sin(phi_4))^2 - ((l_1*sin(phi_1) - l_4*sin(phi_4))^2 + (l_5 - l_1*cos(phi_1) + l_4*cos(phi_4))^2 + l_2^2 - l_3^2)^2 + 4*l_2^2*(l_5 - l_1*cos(phi_1) + l_4*cos(phi_4))^2)^(1/2) - 2*l_2*(l_1*sin(phi_1) - l_4*sin(phi_4)))/((l_1*sin(phi_1) - l_4*sin(phi_4))^2 + (l_5 - l_1*cos(phi_1) + l_4*cos(phi_4))^2 + l_2^2 - l_3^2 + 2*l_2*(l_5 - l_1*cos(phi_1) + l_4*cos(phi_4))))) - l_5/2 + l_1*cos(phi_1)))*(l_2*cos(2*atan(((4*l_2^2*(l_1*sin(phi_1) - l_4*sin(phi_4))^2 - ((l_1*sin(phi_1) - l_4*sin(phi_4))^2 + (l_5 - l_1*cos(phi_1) + l_4*cos(phi_4))^2 + l_2^2 - l_3^2)^2 + 4*l_2^2*(l_5 - l_1*cos(phi_1) + l_4*cos(phi_4))^2)^(1/2) - 2*l_2*(l_1*sin(phi_1) - l_4*sin(phi_4)))/((l_1*sin(phi_1) - l_4*sin(phi_4))^2 + (l_5 - l_1*cos(phi_1) + l_4*cos(phi_4))^2 + l_2^2 - l_3^2 + 2*l_2*(l_5 - l_1*cos(phi_1) + l_4*cos(phi_4))))) - l_5/2 + l_1*cos(phi_1)))/(2*((l_2*sin(2*atan(((4*l_2^2*(l_1*sin(phi_1) - l_4*sin(phi_4))^2 - ((l_1*sin(phi_1) - l_4*sin(phi_4))^2 + (l_5 - l_1*cos(phi_1) + l_4*cos(phi_4))^2 + l_2^2 - l_3^2)^2 + 4*l_2^2*(l_5 - l_1*cos(phi_1) + l_4*cos(phi_4))^2)^(1/2) - 2*l_2*(l_1*sin(phi_1) - l_4*sin(phi_4)))/((l_1*sin(phi_1) - l_4*sin(phi_4))^2 + (l_5 - l_1*cos(phi_1) + l_4*cos(phi_4))^2 + l_2^2 - l_3^2 + 2*l_2*(l_5 - l_1*cos(phi_1) + l_4*cos(phi_4))))) + l_1*sin(phi_1))^2 + (l_2*cos(2*atan(((4*l_2^2*(l_1*sin(phi_1) - l_4*sin(phi_4))^2 - ((l_1*sin(phi_1) - l_4*sin(phi_4))^2 + (l_5 - l_1*cos(phi_1) + l_4*cos(phi_4))^2 + l_2^2 - l_3^2)^2 + 4*l_2^2*(l_5 - l_1*cos(phi_1) + l_4*cos(phi_4))^2)^(1/2) - 2*l_2*(l_1*sin(phi_1) - l_4*sin(phi_4)))/((l_1*sin(phi_1) - l_4*sin(phi_4))^2 + (l_5 - l_1*cos(phi_1) + l_4*cos(phi_4))^2 + l_2^2 - l_3^2 + 2*l_2*(l_5 - l_1*cos(phi_1) + l_4*cos(phi_4))))) - l_5/2 + l_1*cos(phi_1))^2)^(3/2)))/(1 - (l_2*cos(2*atan(((4*l_2^2*(l_1*sin(phi_1) - l_4*sin(phi_4))^2 - ((l_1*sin(phi_1) - l_4*sin(phi_4))^2 + (l_5 - l_1*cos(phi_1) + l_4*cos(phi_4))^2 + l_2^2 - l_3^2)^2 + 4*l_2^2*(l_5 - l_1*cos(phi_1) + l_4*cos(phi_4))^2)^(1/2) - 2*l_2*(l_1*sin(phi_1) - l_4*sin(phi_4)))/((l_1*sin(phi_1) - l_4*sin(phi_4))^2 + (l_5 - l_1*cos(phi_1) + l_4*cos(phi_4))^2 + l_2^2 - l_3^2 + 2*l_2*(l_5 - l_1*cos(phi_1) + l_4*cos(phi_4))))) - l_5/2 + l_1*cos(phi_1))^2/((l_2*sin(2*atan(((4*l_2^2*(l_1*sin(phi_1) - l_4*sin(phi_4))^2 - ((l_1*sin(phi_1) - l_4*sin(phi_4))^2 + (l_5 - l_1*cos(phi_1) + l_4*cos(phi_4))^2 + l_2^2 - l_3^2)^2 + 4*l_2^2*(l_5 - l_1*cos(phi_1) + l_4*cos(phi_4))^2)^(1/2) - 2*l_2*(l_1*sin(phi_1) - l_4*sin(phi_4)))/((l_1*sin(phi_1) - l_4*sin(phi_4))^2 + (l_5 - l_1*cos(phi_1) + l_4*cos(phi_4))^2 + l_2^2 - l_3^2 + 2*l_2*(l_5 - l_1*cos(phi_1) + l_4*cos(phi_4))))) + l_1*sin(phi_1))^2 + (l_2*cos(2*atan(((4*l_2^2*(l_1*sin(phi_1) - l_4*sin(phi_4))^2 - ((l_1*sin(phi_1) - l_4*sin(phi_4))^2 + (l_5 - l_1*cos(phi_1) + l_4*cos(phi_4))^2 + l_2^2 - l_3^2)^2 + 4*l_2^2*(l_5 - l_1*cos(phi_1) + l_4*cos(phi_4))^2)^(1/2) - 2*l_2*(l_1*sin(phi_1) - l_4*sin(phi_4)))/((l_1*sin(phi_1) - l_4*sin(phi_4))^2 + (l_5 - l_1*cos(phi_1) + l_4*cos(phi_4))^2 + l_2^2 - l_3^2 + 2*l_2*(l_5 - l_1*cos(phi_1) + l_4*cos(phi_4))))) - l_5/2 + l_1*cos(phi_1))^2))^(1/2);
J22=((((4*l_2*sin(2*atan(((4*l_2^2*(l_1*sin(phi_1) - l_4*sin(phi_4))^2 - ((l_1*sin(phi_1) - l_4*sin(phi_4))^2 + (l_5 - l_1*cos(phi_1) + l_4*cos(phi_4))^2 + l_2^2 - l_3^2)^2 + 4*l_2^2*(l_5 - l_1*cos(phi_1) + l_4*cos(phi_4))^2)^(1/2) - 2*l_2*(l_1*sin(phi_1) - l_4*sin(phi_4)))/((l_1*sin(phi_1) - l_4*sin(phi_4))^2 + (l_5 - l_1*cos(phi_1) + l_4*cos(phi_4))^2 + l_2^2 - l_3^2 + 2*l_2*(l_5 - l_1*cos(phi_1) + l_4*cos(phi_4)))))*(((8*l_2^2*l_4*cos(phi_4)*(l_1*sin(phi_1) - l_4*sin(phi_4)) - 2*(2*l_4*cos(phi_4)*(l_1*sin(phi_1) - l_4*sin(phi_4)) + 2*l_4*sin(phi_4)*(l_5 - l_1*cos(phi_1) + l_4*cos(phi_4)))*((l_1*sin(phi_1) - l_4*sin(phi_4))^2 + (l_5 - l_1*cos(phi_1) + l_4*cos(phi_4))^2 + l_2^2 - l_3^2) + 8*l_2^2*l_4*sin(phi_4)*(l_5 - l_1*cos(phi_1) + l_4*cos(phi_4)))/(2*(4*l_2^2*(l_1*sin(phi_1) - l_4*sin(phi_4))^2 - ((l_1*sin(phi_1) - l_4*sin(phi_4))^2 + (l_5 - l_1*cos(phi_1) + l_4*cos(phi_4))^2 + l_2^2 - l_3^2)^2 + 4*l_2^2*(l_5 - l_1*cos(phi_1) + l_4*cos(phi_4))^2)^(1/2)) - 2*l_2*l_4*cos(phi_4))/((l_1*sin(phi_1) - l_4*sin(phi_4))^2 + (l_5 - l_1*cos(phi_1) + l_4*cos(phi_4))^2 + l_2^2 - l_3^2 + 2*l_2*(l_5 - l_1*cos(phi_1) + l_4*cos(phi_4))) - (((4*l_2^2*(l_1*sin(phi_1) - l_4*sin(phi_4))^2 - ((l_1*sin(phi_1) - l_4*sin(phi_4))^2 + (l_5 - l_1*cos(phi_1) + l_4*cos(phi_4))^2 + l_2^2 - l_3^2)^2 + 4*l_2^2*(l_5 - l_1*cos(phi_1) + l_4*cos(phi_4))^2)^(1/2) - 2*l_2*(l_1*sin(phi_1) - l_4*sin(phi_4)))*(2*l_2*l_4*sin(phi_4) + 2*l_4*cos(phi_4)*(l_1*sin(phi_1) - l_4*sin(phi_4)) + 2*l_4*sin(phi_4)*(l_5 - l_1*cos(phi_1) + l_4*cos(phi_4))))/((l_1*sin(phi_1) - l_4*sin(phi_4))^2 + (l_5 - l_1*cos(phi_1) + l_4*cos(phi_4))^2 + l_2^2 - l_3^2 + 2*l_2*(l_5 - l_1*cos(phi_1) + l_4*cos(phi_4)))^2)*(l_2*cos(2*atan(((4*l_2^2*(l_1*sin(phi_1) - l_4*sin(phi_4))^2 - ((l_1*sin(phi_1) - l_4*sin(phi_4))^2 + (l_5 - l_1*cos(phi_1) + l_4*cos(phi_4))^2 + l_2^2 - l_3^2)^2 + 4*l_2^2*(l_5 - l_1*cos(phi_1) + l_4*cos(phi_4))^2)^(1/2) - 2*l_2*(l_1*sin(phi_1) - l_4*sin(phi_4)))/((l_1*sin(phi_1) - l_4*sin(phi_4))^2 + (l_5 - l_1*cos(phi_1) + l_4*cos(phi_4))^2 + l_2^2 - l_3^2 + 2*l_2*(l_5 - l_1*cos(phi_1) + l_4*cos(phi_4))))) - l_5/2 + l_1*cos(phi_1)))/(((4*l_2^2*(l_1*sin(phi_1) - l_4*sin(phi_4))^2 - ((l_1*sin(phi_1) - l_4*sin(phi_4))^2 + (l_5 - l_1*cos(phi_1) + l_4*cos(phi_4))^2 + l_2^2 - l_3^2)^2 + 4*l_2^2*(l_5 - l_1*cos(phi_1) + l_4*cos(phi_4))^2)^(1/2) - 2*l_2*(l_1*sin(phi_1) - l_4*sin(phi_4)))^2/((l_1*sin(phi_1) - l_4*sin(phi_4))^2 + (l_5 - l_1*cos(phi_1) + l_4*cos(phi_4))^2 + l_2^2 - l_3^2 + 2*l_2*(l_5 - l_1*cos(phi_1) + l_4*cos(phi_4)))^2 + 1) - (4*l_2*cos(2*atan(((4*l_2^2*(l_1*sin(phi_1) - l_4*sin(phi_4))^2 - ((l_1*sin(phi_1) - l_4*sin(phi_4))^2 + (l_5 - l_1*cos(phi_1) + l_4*cos(phi_4))^2 + l_2^2 - l_3^2)^2 + 4*l_2^2*(l_5 - l_1*cos(phi_1) + l_4*cos(phi_4))^2)^(1/2) - 2*l_2*(l_1*sin(phi_1) - l_4*sin(phi_4)))/((l_1*sin(phi_1) - l_4*sin(phi_4))^2 + (l_5 - l_1*cos(phi_1) + l_4*cos(phi_4))^2 + l_2^2 - l_3^2 + 2*l_2*(l_5 - l_1*cos(phi_1) + l_4*cos(phi_4)))))*(l_2*sin(2*atan(((4*l_2^2*(l_1*sin(phi_1) - l_4*sin(phi_4))^2 - ((l_1*sin(phi_1) - l_4*sin(phi_4))^2 + (l_5 - l_1*cos(phi_1) + l_4*cos(phi_4))^2 + l_2^2 - l_3^2)^2 + 4*l_2^2*(l_5 - l_1*cos(phi_1) + l_4*cos(phi_4))^2)^(1/2) - 2*l_2*(l_1*sin(phi_1) - l_4*sin(phi_4)))/((l_1*sin(phi_1) - l_4*sin(phi_4))^2 + (l_5 - l_1*cos(phi_1) + l_4*cos(phi_4))^2 + l_2^2 - l_3^2 + 2*l_2*(l_5 - l_1*cos(phi_1) + l_4*cos(phi_4))))) + l_1*sin(phi_1))*(((8*l_2^2*l_4*cos(phi_4)*(l_1*sin(phi_1) - l_4*sin(phi_4)) - 2*(2*l_4*cos(phi_4)*(l_1*sin(phi_1) - l_4*sin(phi_4)) + 2*l_4*sin(phi_4)*(l_5 - l_1*cos(phi_1) + l_4*cos(phi_4)))*((l_1*sin(phi_1) - l_4*sin(phi_4))^2 + (l_5 - l_1*cos(phi_1) + l_4*cos(phi_4))^2 + l_2^2 - l_3^2) + 8*l_2^2*l_4*sin(phi_4)*(l_5 - l_1*cos(phi_1) + l_4*cos(phi_4)))/(2*(4*l_2^2*(l_1*sin(phi_1) - l_4*sin(phi_4))^2 - ((l_1*sin(phi_1) - l_4*sin(phi_4))^2 + (l_5 - l_1*cos(phi_1) + l_4*cos(phi_4))^2 + l_2^2 - l_3^2)^2 + 4*l_2^2*(l_5 - l_1*cos(phi_1) + l_4*cos(phi_4))^2)^(1/2)) - 2*l_2*l_4*cos(phi_4))/((l_1*sin(phi_1) - l_4*sin(phi_4))^2 + (l_5 - l_1*cos(phi_1) + l_4*cos(phi_4))^2 + l_2^2 - l_3^2 + 2*l_2*(l_5 - l_1*cos(phi_1) + l_4*cos(phi_4))) - (((4*l_2^2*(l_1*sin(phi_1) - l_4*sin(phi_4))^2 - ((l_1*sin(phi_1) - l_4*sin(phi_4))^2 + (l_5 - l_1*cos(phi_1) + l_4*cos(phi_4))^2 + l_2^2 - l_3^2)^2 + 4*l_2^2*(l_5 - l_1*cos(phi_1) + l_4*cos(phi_4))^2)^(1/2) - 2*l_2*(l_1*sin(phi_1) - l_4*sin(phi_4)))*(2*l_2*l_4*sin(phi_4) + 2*l_4*cos(phi_4)*(l_1*sin(phi_1) - l_4*sin(phi_4)) + 2*l_4*sin(phi_4)*(l_5 - l_1*cos(phi_1) + l_4*cos(phi_4))))/((l_1*sin(phi_1) - l_4*sin(phi_4))^2 + (l_5 - l_1*cos(phi_1) + l_4*cos(phi_4))^2 + l_2^2 - l_3^2 + 2*l_2*(l_5 - l_1*cos(phi_1) + l_4*cos(phi_4)))^2))/(((4*l_2^2*(l_1*sin(phi_1) - l_4*sin(phi_4))^2 - ((l_1*sin(phi_1) - l_4*sin(phi_4))^2 + (l_5 - l_1*cos(phi_1) + l_4*cos(phi_4))^2 + l_2^2 - l_3^2)^2 + 4*l_2^2*(l_5 - l_1*cos(phi_1) + l_4*cos(phi_4))^2)^(1/2) - 2*l_2*(l_1*sin(phi_1) - l_4*sin(phi_4)))^2/((l_1*sin(phi_1) - l_4*sin(phi_4))^2 + (l_5 - l_1*cos(phi_1) + l_4*cos(phi_4))^2 + l_2^2 - l_3^2 + 2*l_2*(l_5 - l_1*cos(phi_1) + l_4*cos(phi_4)))^2 + 1))*(l_2*cos(2*atan(((4*l_2^2*(l_1*sin(phi_1) - l_4*sin(phi_4))^2 - ((l_1*sin(phi_1) - l_4*sin(phi_4))^2 + (l_5 - l_1*cos(phi_1) + l_4*cos(phi_4))^2 + l_2^2 - l_3^2)^2 + 4*l_2^2*(l_5 - l_1*cos(phi_1) + l_4*cos(phi_4))^2)^(1/2) - 2*l_2*(l_1*sin(phi_1) - l_4*sin(phi_4)))/((l_1*sin(phi_1) - l_4*sin(phi_4))^2 + (l_5 - l_1*cos(phi_1) + l_4*cos(phi_4))^2 + l_2^2 - l_3^2 + 2*l_2*(l_5 - l_1*cos(phi_1) + l_4*cos(phi_4))))) - l_5/2 + l_1*cos(phi_1)))/(2*((l_2*sin(2*atan(((4*l_2^2*(l_1*sin(phi_1) - l_4*sin(phi_4))^2 - ((l_1*sin(phi_1) - l_4*sin(phi_4))^2 + (l_5 - l_1*cos(phi_1) + l_4*cos(phi_4))^2 + l_2^2 - l_3^2)^2 + 4*l_2^2*(l_5 - l_1*cos(phi_1) + l_4*cos(phi_4))^2)^(1/2) - 2*l_2*(l_1*sin(phi_1) - l_4*sin(phi_4)))/((l_1*sin(phi_1) - l_4*sin(phi_4))^2 + (l_5 - l_1*cos(phi_1) + l_4*cos(phi_4))^2 + l_2^2 - l_3^2 + 2*l_2*(l_5 - l_1*cos(phi_1) + l_4*cos(phi_4))))) + l_1*sin(phi_1))^2 + (l_2*cos(2*atan(((4*l_2^2*(l_1*sin(phi_1) - l_4*sin(phi_4))^2 - ((l_1*sin(phi_1) - l_4*sin(phi_4))^2 + (l_5 - l_1*cos(phi_1) + l_4*cos(phi_4))^2 + l_2^2 - l_3^2)^2 + 4*l_2^2*(l_5 - l_1*cos(phi_1) + l_4*cos(phi_4))^2)^(1/2) - 2*l_2*(l_1*sin(phi_1) - l_4*sin(phi_4)))/((l_1*sin(phi_1) - l_4*sin(phi_4))^2 + (l_5 - l_1*cos(phi_1) + l_4*cos(phi_4))^2 + l_2^2 - l_3^2 + 2*l_2*(l_5 - l_1*cos(phi_1) + l_4*cos(phi_4))))) - l_5/2 + l_1*cos(phi_1))^2)^(3/2)) - (2*l_2*sin(2*atan(((4*l_2^2*(l_1*sin(phi_1) - l_4*sin(phi_4))^2 - ((l_1*sin(phi_1) - l_4*sin(phi_4))^2 + (l_5 - l_1*cos(phi_1) + l_4*cos(phi_4))^2 + l_2^2 - l_3^2)^2 + 4*l_2^2*(l_5 - l_1*cos(phi_1) + l_4*cos(phi_4))^2)^(1/2) - 2*l_2*(l_1*sin(phi_1) - l_4*sin(phi_4)))/((l_1*sin(phi_1) - l_4*sin(phi_4))^2 + (l_5 - l_1*cos(phi_1) + l_4*cos(phi_4))^2 + l_2^2 - l_3^2 + 2*l_2*(l_5 - l_1*cos(phi_1) + l_4*cos(phi_4)))))*(((8*l_2^2*l_4*cos(phi_4)*(l_1*sin(phi_1) - l_4*sin(phi_4)) - 2*(2*l_4*cos(phi_4)*(l_1*sin(phi_1) - l_4*sin(phi_4)) + 2*l_4*sin(phi_4)*(l_5 - l_1*cos(phi_1) + l_4*cos(phi_4)))*((l_1*sin(phi_1) - l_4*sin(phi_4))^2 + (l_5 - l_1*cos(phi_1) + l_4*cos(phi_4))^2 + l_2^2 - l_3^2) + 8*l_2^2*l_4*sin(phi_4)*(l_5 - l_1*cos(phi_1) + l_4*cos(phi_4)))/(2*(4*l_2^2*(l_1*sin(phi_1) - l_4*sin(phi_4))^2 - ((l_1*sin(phi_1) - l_4*sin(phi_4))^2 + (l_5 - l_1*cos(phi_1) + l_4*cos(phi_4))^2 + l_2^2 - l_3^2)^2 + 4*l_2^2*(l_5 - l_1*cos(phi_1) + l_4*cos(phi_4))^2)^(1/2)) - 2*l_2*l_4*cos(phi_4))/((l_1*sin(phi_1) - l_4*sin(phi_4))^2 + (l_5 - l_1*cos(phi_1) + l_4*cos(phi_4))^2 + l_2^2 - l_3^2 + 2*l_2*(l_5 - l_1*cos(phi_1) + l_4*cos(phi_4))) - (((4*l_2^2*(l_1*sin(phi_1) - l_4*sin(phi_4))^2 - ((l_1*sin(phi_1) - l_4*sin(phi_4))^2 + (l_5 - l_1*cos(phi_1) + l_4*cos(phi_4))^2 + l_2^2 - l_3^2)^2 + 4*l_2^2*(l_5 - l_1*cos(phi_1) + l_4*cos(phi_4))^2)^(1/2) - 2*l_2*(l_1*sin(phi_1) - l_4*sin(phi_4)))*(2*l_2*l_4*sin(phi_4) + 2*l_4*cos(phi_4)*(l_1*sin(phi_1) - l_4*sin(phi_4)) + 2*l_4*sin(phi_4)*(l_5 - l_1*cos(phi_1) + l_4*cos(phi_4))))/((l_1*sin(phi_1) - l_4*sin(phi_4))^2 + (l_5 - l_1*cos(phi_1) + l_4*cos(phi_4))^2 + l_2^2 - l_3^2 + 2*l_2*(l_5 - l_1*cos(phi_1) + l_4*cos(phi_4)))^2))/(((l_2*sin(2*atan(((4*l_2^2*(l_1*sin(phi_1) - l_4*sin(phi_4))^2 - ((l_1*sin(phi_1) - l_4*sin(phi_4))^2 + (l_5 - l_1*cos(phi_1) + l_4*cos(phi_4))^2 + l_2^2 - l_3^2)^2 + 4*l_2^2*(l_5 - l_1*cos(phi_1) + l_4*cos(phi_4))^2)^(1/2) - 2*l_2*(l_1*sin(phi_1) - l_4*sin(phi_4)))/((l_1*sin(phi_1) - l_4*sin(phi_4))^2 + (l_5 - l_1*cos(phi_1) + l_4*cos(phi_4))^2 + l_2^2 - l_3^2 + 2*l_2*(l_5 - l_1*cos(phi_1) + l_4*cos(phi_4))))) + l_1*sin(phi_1))^2 + (l_2*cos(2*atan(((4*l_2^2*(l_1*sin(phi_1) - l_4*sin(phi_4))^2 - ((l_1*sin(phi_1) - l_4*sin(phi_4))^2 + (l_5 - l_1*cos(phi_1) + l_4*cos(phi_4))^2 + l_2^2 - l_3^2)^2 + 4*l_2^2*(l_5 - l_1*cos(phi_1) + l_4*cos(phi_4))^2)^(1/2) - 2*l_2*(l_1*sin(phi_1) - l_4*sin(phi_4)))/((l_1*sin(phi_1) - l_4*sin(phi_4))^2 + (l_5 - l_1*cos(phi_1) + l_4*cos(phi_4))^2 + l_2^2 - l_3^2 + 2*l_2*(l_5 - l_1*cos(phi_1) + l_4*cos(phi_4))))) - l_5/2 + l_1*cos(phi_1))^2)^(1/2)*(((4*l_2^2*(l_1*sin(phi_1) - l_4*sin(phi_4))^2 - ((l_1*sin(phi_1) - l_4*sin(phi_4))^2 + (l_5 - l_1*cos(phi_1) + l_4*cos(phi_4))^2 + l_2^2 - l_3^2)^2 + 4*l_2^2*(l_5 - l_1*cos(phi_1) + l_4*cos(phi_4))^2)^(1/2) - 2*l_2*(l_1*sin(phi_1) - l_4*sin(phi_4)))^2/((l_1*sin(phi_1) - l_4*sin(phi_4))^2 + (l_5 - l_1*cos(phi_1) + l_4*cos(phi_4))^2 + l_2^2 - l_3^2 + 2*l_2*(l_5 - l_1*cos(phi_1) + l_4*cos(phi_4)))^2 + 1)))/(1 - (l_2*cos(2*atan(((4*l_2^2*(l_1*sin(phi_1) - l_4*sin(phi_4))^2 - ((l_1*sin(phi_1) - l_4*sin(phi_4))^2 + (l_5 - l_1*cos(phi_1) + l_4*cos(phi_4))^2 + l_2^2 - l_3^2)^2 + 4*l_2^2*(l_5 - l_1*cos(phi_1) + l_4*cos(phi_4))^2)^(1/2) - 2*l_2*(l_1*sin(phi_1) - l_4*sin(phi_4)))/((l_1*sin(phi_1) - l_4*sin(phi_4))^2 + (l_5 - l_1*cos(phi_1) + l_4*cos(phi_4))^2 + l_2^2 - l_3^2 + 2*l_2*(l_5 - l_1*cos(phi_1) + l_4*cos(phi_4))))) - l_5/2 + l_1*cos(phi_1))^2/((l_2*sin(2*atan(((4*l_2^2*(l_1*sin(phi_1) - l_4*sin(phi_4))^2 - ((l_1*sin(phi_1) - l_4*sin(phi_4))^2 + (l_5 - l_1*cos(phi_1) + l_4*cos(phi_4))^2 + l_2^2 - l_3^2)^2 + 4*l_2^2*(l_5 - l_1*cos(phi_1) + l_4*cos(phi_4))^2)^(1/2) - 2*l_2*(l_1*sin(phi_1) - l_4*sin(phi_4)))/((l_1*sin(phi_1) - l_4*sin(phi_4))^2 + (l_5 - l_1*cos(phi_1) + l_4*cos(phi_4))^2 + l_2^2 - l_3^2 + 2*l_2*(l_5 - l_1*cos(phi_1) + l_4*cos(phi_4))))) + l_1*sin(phi_1))^2 + (l_2*cos(2*atan(((4*l_2^2*(l_1*sin(phi_1) - l_4*sin(phi_4))^2 - ((l_1*sin(phi_1) - l_4*sin(phi_4))^2 + (l_5 - l_1*cos(phi_1) + l_4*cos(phi_4))^2 + l_2^2 - l_3^2)^2 + 4*l_2^2*(l_5 - l_1*cos(phi_1) + l_4*cos(phi_4))^2)^(1/2) - 2*l_2*(l_1*sin(phi_1) - l_4*sin(phi_4)))/((l_1*sin(phi_1) - l_4*sin(phi_4))^2 + (l_5 - l_1*cos(phi_1) + l_4*cos(phi_4))^2 + l_2^2 - l_3^2 + 2*l_2*(l_5 - l_1*cos(phi_1) + l_4*cos(phi_4))))) - l_5/2 + l_1*cos(phi_1))^2))^(1/2);

T1=J11*F+J21*Tp;
T2=J12*F+J22*Tp;

== matlab function Model/右腿数据处理/MATLAB Function ==
  data: phi_1 input; L_0 output; phi_4 input; phi_0 output; phi_2 output
function [L_0,phi_0,phi_2]= fcn(phi_1,phi_4)

l_1=0.15;
l_2=0.27;
l_3=0.27;
l_4=0.15;
l_5=0.15;

L_0=((l_2*sin(2*atan(((4*l_2^2*(l_1*sin(phi_1) - l_4*sin(phi_4))^2 - ((l_1*sin(phi_1) - l_4*sin(phi_4))^2 + (l_5 - l_1*cos(phi_1) + l_4*cos(phi_4))^2 + l_2^2 - l_3^2)^2 + 4*l_2^2*(l_5 - l_1*cos(phi_1) + l_4*cos(phi_4))^2)^(1/2) - 2*l_2*(l_1*sin(phi_1) - l_4*sin(phi_4)))/((l_1*sin(phi_1) - l_4*sin(phi_4))^2 + (l_5 - l_1*cos(phi_1) + l_4*cos(phi_4))^2 + l_2^2 - l_3^2 + 2*l_2*(l_5 - l_1*cos(phi_1) + l_4*cos(phi_4))))) + l_1*sin(phi_1))^2 + (l_2*cos(2*atan(((4*l_2^2*(l_1*sin(phi_1) - l_4*sin(phi_4))^2 - ((l_1*sin(phi_1) - l_4*sin(phi_4))^2 + (l_5 - l_1*cos(phi_1) + l_4*cos(phi_4))^2 + l_2^2 - l_3^2)^2 + 4*l_2^2*(l_5 - l_1*cos(phi_1) + l_4*cos(phi_4))^2)^(1/2) - 2*l_2*(l_1*sin(phi_1) - l_4*sin(phi_4)))/((l_1*sin(phi_1) - l_4*sin(phi_4))^2 + (l_5 - l_1*cos(phi_1) + l_4*cos(phi_4))^2 + l_2^2 - l_3^2 + 2*l_2*(l_5 - l_1*cos(phi_1) + l_4*cos(phi_4))))) - l_5/2 + l_1*cos(phi_1))^2)^(1/2);
phi_0=acos((l_2*cos(2*atan(((4*l_2^2*(l_1*sin(phi_1) - l_4*sin(phi_4))^2 - ((l_1*sin(phi_1) - l_4*sin(phi_4))^2 + (l_5 - l_1*cos(phi_1) + l_4*cos(phi_4))^2 + l_2^2 - l_3^2)^2 + 4*l_2^2*(l_5 - l_1*cos(phi_1) + l_4*cos(phi_4))^2)^(1/2) - 2*l_2*(l_1*sin(phi_1) - l_4*sin(phi_4)))/((l_1*sin(phi_1) - l_4*sin(phi_4))^2 + (l_5 - l_1*cos(phi_1) + l_4*cos(phi_4))^2 + l_2^2 - l_3^2 + 2*l_2*(l_5 - l_1*cos(phi_1) + l_4*cos(phi_4))))) - l_5/2 + l_1*cos(phi_1))/((l_2*sin(2*atan(((4*l_2^2*(l_1*sin(phi_1) - l_4*sin(phi_4))^2 - ((l_1*sin(phi_1) - l_4*sin(phi_4))^2 + (l_5 - l_1*cos(phi_1) + l_4*cos(phi_4))^2 + l_2^2 - l_3^2)^2 + 4*l_2^2*(l_5 - l_1*cos(phi_1) + l_4*cos(phi_4))^2)^(1/2) - 2*l_2*(l_1*sin(phi_1) - l_4*sin(phi_4)))/((l_1*sin(phi_1) - l_4*sin(phi_4))^2 + (l_5 - l_1*cos(phi_1) + l_4*cos(phi_4))^2 + l_2^2 - l_3^2 + 2*l_2*(l_5 - l_1*cos(phi_1) + l_4*cos(phi_4))))) + l_1*sin(phi_1))^2 + (l_2*cos(2*atan(((4*l_2^2*(l_1*sin(phi_1) - l_4*sin(phi_4))^2 - ((l_1*sin(phi_1) - l_4*sin(phi_4))^2 + (l_5 - l_1*cos(phi_1) + l_4*cos(phi_4))^2 + l_2^2 - l_3^2)^2 + 4*l_2^2*(l_5 - l_1*cos(phi_1) + l_4*cos(phi_4))^2)^(1/2) - 2*l_2*(l_1*sin(phi_1) - l_4*sin(phi_4)))/((l_1*sin(phi_1) - l_4*sin(phi_4))^2 + (l_5 - l_1*cos(phi_1) + l_4*cos(phi_4))^2 + l_2^2 - l_3^2 + 2*l_2*(l_5 - l_1*cos(phi_1) + l_4*cos(phi_4))))) - l_5/2 + l_1*cos(phi_1))^2)^(1/2));
phi_2=2*atan(((4*l_2^2*(l_1*sin(phi_1) - l_4*sin(phi_4))^2 - ((l_1*sin(phi_1) - l_4*sin(phi_4))^2 + (l_5 - l_1*cos(phi_1) + l_4*cos(phi_4))^2 + l_2^2 - l_3^2)^2 + 4*l_2^2*(l_5 - l_1*cos(phi_1) + l_4*cos(phi_4))^2)^(1/2) - 2*l_2*(l_1*sin(phi_1) - l_4*sin(phi_4)))/((l_1*sin(phi_1) - l_4*sin(phi_4))^2 + (l_5 - l_1*cos(phi_1) + l_4*cos(phi_4))^2 + l_2^2 - l_3^2 + 2*l_2*(l_5 - l_1*cos(phi_1) + l_4*cos(phi_4))));

== matlab function Model/左腿数据处理/MATLAB Function ==
  data: phi_1 input; L_0 output; phi_4 input; phi_0 output; phi_2 output
function [L_0,phi_0,phi_2]= fcn(phi_1,phi_4)

l_1=0.15;
l_2=0.27;
l_3=0.27;
l_4=0.15;
l_5=0.15;

L_0=((l_2*sin(2*atan(((4*l_2^2*(l_1*sin(phi_1) - l_4*sin(phi_4))^2 - ((l_1*sin(phi_1) - l_4*sin(phi_4))^2 + (l_5 - l_1*cos(phi_1) + l_4*cos(phi_4))^2 + l_2^2 - l_3^2)^2 + 4*l_2^2*(l_5 - l_1*cos(phi_1) + l_4*cos(phi_4))^2)^(1/2) - 2*l_2*(l_1*sin(phi_1) - l_4*sin(phi_4)))/((l_1*sin(phi_1) - l_4*sin(phi_4))^2 + (l_5 - l_1*cos(phi_1) + l_4*cos(phi_4))^2 + l_2^2 - l_3^2 + 2*l_2*(l_5 - l_1*cos(phi_1) + l_4*cos(phi_4))))) + l_1*sin(phi_1))^2 + (l_2*cos(2*atan(((4*l_2^2*(l_1*sin(phi_1) - l_4*sin(phi_4))^2 - ((l_1*sin(phi_1) - l_4*sin(phi_4))^2 + (l_5 - l_1*cos(phi_1) + l_4*cos(phi_4))^2 + l_2^2 - l_3^2)^2 + 4*l_2^2*(l_5 - l_1*cos(phi_1) + l_4*cos(phi_4))^2)^(1/2) - 2*l_2*(l_1*sin(phi_1) - l_4*sin(phi_4)))/((l_1*sin(phi_1) - l_4*sin(phi_4))^2 + (l_5 - l_1*cos(phi_1) + l_4*cos(phi_4))^2 + l_2^2 - l_3^2 + 2*l_2*(l_5 - l_1*cos(phi_1) + l_4*cos(phi_4))))) - l_5/2 + l_1*cos(phi_1))^2)^(1/2);
phi_0=acos((l_2*cos(2*atan(((4*l_2^2*(l_1*sin(phi_1) - l_4*sin(phi_4))^2 - ((l_1*sin(phi_1) - l_4*sin(phi_4))^2 + (l_5 - l_1*cos(phi_1) + l_4*cos(phi_4))^2 + l_2^2 - l_3^2)^2 + 4*l_2^2*(l_5 - l_1*cos(phi_1) + l_4*cos(phi_4))^2)^(1/2) - 2*l_2*(l_1*sin(phi_1) - l_4*sin(phi_4)))/((l_1*sin(phi_1) - l_4*sin(phi_4))^2 + (l_5 - l_1*cos(phi_1) + l_4*cos(phi_4))^2 + l_2^2 - l_3^2 + 2*l_2*(l_5 - l_1*cos(phi_1) + l_4*cos(phi_4))))) - l_5/2 + l_1*cos(phi_1))/((l_2*sin(2*atan(((4*l_2^2*(l_1*sin(phi_1) - l_4*sin(phi_4))^2 - ((l_1*sin(phi_1) - l_4*sin(phi_4))^2 + (l_5 - l_1*cos(phi_1) + l_4*cos(phi_4))^2 + l_2^2 - l_3^2)^2 + 4*l_2^2*(l_5 - l_1*cos(phi_1) + l_4*cos(phi_4))^2)^(1/2) - 2*l_2*(l_1*sin(phi_1) - l_4*sin(phi_4)))/((l_1*sin(phi_1) - l_4*sin(phi_4))^2 + (l_5 - l_1*cos(phi_1) + l_4*cos(phi_4))^2 + l_2^2 - l_3^2 + 2*l_2*(l_5 - l_1*cos(phi_1) + l_4*cos(phi_4))))) + l_1*sin(phi_1))^2 + (l_2*cos(2*atan(((4*l_2^2*(l_1*sin(phi_1) - l_4*sin(phi_4))^2 - ((l_1*sin(phi_1) - l_4*sin(phi_4))^2 + (l_5 - l_1*cos(phi_1) + l_4*cos(phi_4))^2 + l_2^2 - l_3^2)^2 + 4*l_2^2*(l_5 - l_1*cos(phi_1) + l_4*cos(phi_4))^2)^(1/2) - 2*l_2*(l_1*sin(phi_1) - l_4*sin(phi_4)))/((l_1*sin(phi_1) - l_4*sin(phi_4))^2 + (l_5 - l_1*cos(phi_1) + l_4*cos(phi_4))^2 + l_2^2 - l_3^2 + 2*l_2*(l_5 - l_1*cos(phi_1) + l_4*cos(phi_4))))) - l_5/2 + l_1*cos(phi_1))^2)^(1/2));
phi_2=2*atan(((4*l_2^2*(l_1*sin(phi_1) - l_4*sin(phi_4))^2 - ((l_1*sin(phi_1) - l_4*sin(phi_4))^2 + (l_5 - l_1*cos(phi_1) + l_4*cos(phi_4))^2 + l_2^2 - l_3^2)^2 + 4*l_2^2*(l_5 - l_1*cos(phi_1) + l_4*cos(phi_4))^2)^(1/2) - 2*l_2*(l_1*sin(phi_1) - l_4*sin(phi_4)))/((l_1*sin(phi_1) - l_4*sin(phi_4))^2 + (l_5 - l_1*cos(phi_1) + l_4*cos(phi_4))^2 + l_2^2 - l_3^2 + 2*l_2*(l_5 - l_1*cos(phi_1) + l_4*cos(phi_4))));
